simulink model "bic_yutong"  (R2018a)
settings: Solver=FixedStepAuto  StartTime=0.0  StopTime=10.0  FixedStep=Ts  RelTol=1e-3  EnableMultiTasking=on
libraries: simulink x1
settings Model: Creator=Administrator  LastModifiedBy=Administrator
settings DataIOCC: LimitDataPoints=on  SaveFormat=Array
settings OptimizationCC: LifeSpan=inf
settings DebuggingCC: SolverPrmCheckMsg=warning  SFUnexpectedBacktrackingDiag=warning  SFNoUnconditionalDefaultTransitionDiag=warning  SFExecutionAtInitializationDiag=none
settings HardwareCC: ProdBitPerPointer=32  ProdBitPerSizeT=32  ProdBitPerPtrDiffT=32  ProdLargestAtomicFloat=None  ProdIntDivRoundTo=Undefined  ProdEndianess=Unspecified  ProdWordSize=32  ProdHWDeviceType=32-bit Generic
settings ModelReferenceCC: PropagateSignalLabelsOutOfModel=off
settings CodeAppCC: StateflowObjectComments=on
settings GRTTargetCC: TargetLangStandard=C89/C90 (ANSI)  GeneratePreprocessorConditionals=Disable all
settings ConfigComp: CovMetricSettings=dw  CovHtmlReporting=on  CovSaveCumulativeToWorkspaceVar=on  CovSaveSingleToWorkspaceVar=on  CovExternalEMLEnable=off  CovSFcnEnable=off

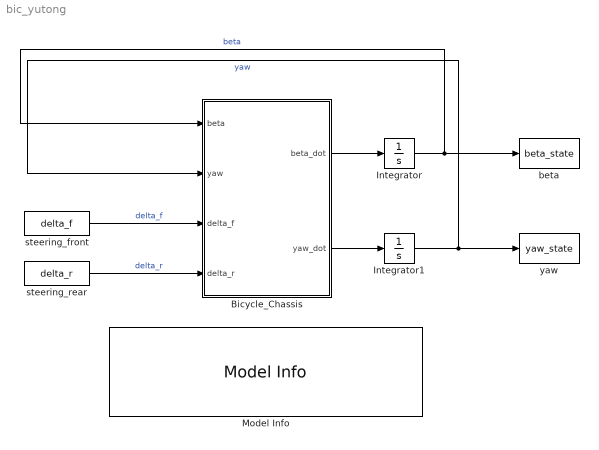
== system bic_yutong ==
  " Bicycle_Chassis" : MATLAB Function  TreatAsAtomicUnit=on
  Integrator : Integrator
  Integrator1 : Integrator
  Model Info : simulink/Model-Wide Utilities/Model Info  Frame=on  DisplayStringWithTags=|  HorizontalTextAlignment=Left  LeftAlignmentValue=0.02
      | Model Info
      | 
      | [delta_f] is the steering angle on the front wheels.
  beta : ToWorkspace  VariableName=beta_state  SampleTime=-1
  steering_front : FromWorkspace  VariableName=delta_f  SampleTime=0
  steering_rear : FromWorkspace  VariableName=delta_r  SampleTime=0
  yaw : ToWorkspace  VariableName=yaw_state  SampleTime=-1
  wires:
  steering_front/1 -> " Bicycle_Chassis"/3(delta_f)  "delta_f"
  steering_rear/1 -> " Bicycle_Chassis"/4(delta_r)  "delta_r"
  " Bicycle_Chassis"/1(beta_dot) -> Integrator/1
  " Bicycle_Chassis"/2(yaw_dot) -> Integrator1/1
  Integrator1/1 -> yaw/1, " Bicycle_Chassis"/2(yaw)  "yaw"
  Integrator/1 -> beta/1, " Bicycle_Chassis"/1(beta)  "beta"

== matlab function bic_yutong/ Bicycle_Chassis ==
  data: beta input; yaw input; delta_f input; beta_dot output; delta_r input; yaw_dot output
function [beta_dot, yaw_dot]   = bicycle(beta, yaw ,delta_f,delta_r)

X = [beta, yaw]';
U = [delta_f,delta_r]';

Cf =  13000;
Cr =  13000;
M =  1600;
lr  =  1.4 ;
lf  =  1.6;
Iz =  3600;

V  = 2; %m/s,  assume the constant speed 
Vx = cos(beta)*V;
% 
a11 = -2*(Cf+Cr)/(M*Vx);
a12 = -(1+(2*Cf*lf-2*Cr*lr)/(M*Vx^2));
a21 = -2*(Cf*lf - Cr*lr)/Iz;
a22 = -2*(Cf*lf^2+Cr*lr^2)/(Iz*Vx);

A = [a11, a12; a21, a22];

b11 = 2*Cf/(M*Vx);
b12 =  2*Cr/(M*Vx);
b21 = 2*Cf*lf/Iz;
b22 = -2*Cr*lr/Iz;

B = [b11, b12; b21, b22];

X_dot = A*X +B*U;

beta_dot = X_dot(1);
yaw_dot = X_dot(2);

end
